simulink model "MinSegShield_Demo_M2V3"  (R2013a)
settings: Solver=FixedStepDiscrete  SolverMode=SingleTasking  StartTime=0.0  StopTime=inf  FixedStep=.1  RelTol=1e-3
libraries: arduinolib x5, MinSegLibrary_M2V3 x2
settings Model: SimulationMode=external  ExtModeTrigDuration=2  Creator=Alec  LastModifiedBy=hurstj
settings OptimizationCC: ExpressionDepthLimit=2147483647  OptimizeModelRefInitCode=on  LifeSpan=1
settings DebuggingCC: SolverPrmCheckMsg=none  StrictBusMsg=Warning
settings HardwareCC: ProdBitPerInt=16  ProdBitPerPointer=8  ProdIntDivRoundTo=Zero  ProdEndianess=LittleEndian  ProdWordSize=8  ProdHWDeviceType=Atmel->AVR
settings RTWCC: SystemTargetFile=realtime.tlc  GenerateMakefile=off  TemplateMakefile=realtime.tmf  Description=Real-Time Toolbox  RTWVerbose=off  ProcessScript=realtime_make_rtw_hook
settings CodeAppCC: CustomSymbolStrType=$N$R$M  InternalIdentifier=Classic
settings STFCustomTargetCC: TargetLibSuffix=.a  GenerateSampleERTMain=on  ERTCustomFileBanners=on  SupportNonInlinedSFcns=off  SupportVariableSizeSignals=on  MATLABClassNameForMDSCustomization=Simulink.SoftwareTarget.ERTCustomization  SystemTargetFile=realtime.tlc
settings ERTTargetCC: ParMdlRefBuildCompliant=off  CompOptLevelCompliant=off  ConcurrentExecutionCompliant=off  CombineOutputUpdateFcns=off  ERTFirstTimeCompliant=off  SupportContinuousTime=on  SupportVariableSizeSignals=on  ModelStepFunctionPrototypeControlCompliant=off  CPPClassGenCompliant=off  ExtMode=on  ExtModeTransport=3  ExtModeMexFile=ext_serial_win32_comm  ExtModeMexArgs=0 68 115200  ERTSrcFileBannerTemplate=realtime_code_template.cgt  ERTHdrFileBannerTemplate=realtime_code_template.cgt  ERTDataSrcFileTemplate=realtime_code_template.cgt  ERTDataHdrFileTemplate=realtime_code_template.cgt  ERTCustomFileTemplate=realtime_file_process.tlc

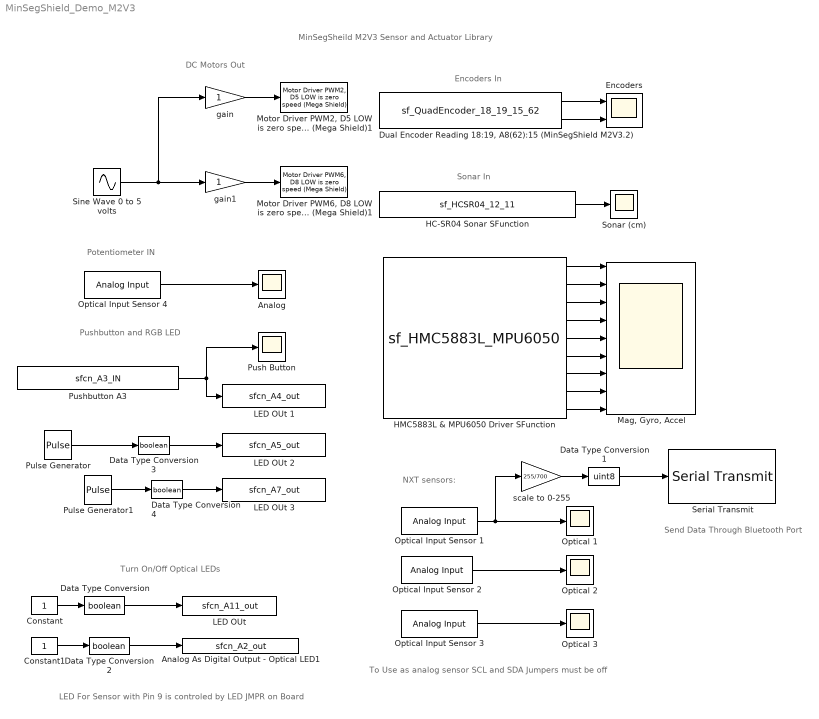
== system MinSegShield_Demo_M2V3 ==
  note: LED For Sensor with Pin 9
      |  is controled by LED JMPR on Board
  note: Turn On/Off Optical LEDs
  note: Send Data Through Bluetooth Port
  note: To Use as analog sensor SCL and SDA Jumpers must be off
  note: Potentiometer IN
  note: Pushbutton and RGB LED
  note: DC Motors Out
  note: Encoders In
  note: Sonar In
  note: NXT sensors:
  note: MinSegSheild M2V3 Sensor and Actuator Library
  Analog : Scope
      settings: TimeRange=30  YMin=0  YMax=1000  SaveName=ScopeData6
  Analog As Digital Output - Optical LED1 : S-Function  InitFcn=try, set_param(gcb,'FunctionName','sfcn_A2_out'), end  FunctionName=sfcn_A2_out  Parameters=uint8(12)  SFunctionModules=sfcn_A2_out_wrapper  EnableBusSupport=off  mask(S-Function Builder){}
      mask init:
      | val = [[.9  0.75 0.75 1 1 .9 .9 1]',[1 1 0.75 0.75 .9 .9 1 .9]'];try , sys = get_param(gcb,'SfunBuilderFcnName');if isempty(sys), sys = get_param(gcb,'FunctionName'); end,catch, sys = get_param(gcb,'FunctionName'); end
      settings: CopyFcn=set_param(gcbh,'LinkStatus','none')  PreSaveFcn=try, set_param(gcb,'FunctionName','sfcn_A2_out'), end  OpenFcn=sfunctionwizard(gcbh)
      mask Display: plot(val(:,1),val(:,2)),disp(sys), port_label('input',1,'in')
  Constant : Constant  SampleTime=-1
  Constant1 : Constant  SampleTime=-1
  Data Type Conversion{,2..4} (4 alike) : DataTypeConversion  OutDataTypeStr=boolean
  Data Type Conversion1 : DataTypeConversion  OutDataTypeStr=uint8
  "Dual Encoder Reading 18:19, A8(62):15 (MinSegShield M2V3.2) " : S-Function  InitFcn=try, set_param(gcb,'FunctionName','sf_QuadEncoder_18_19_15_62'), end  FunctionName=sf_QuadEncoder_18_19_15_62  Parameters=uint8([0 1]),uint8([18 62]),uint8([19 15])  SFunctionModules=sf_QuadEncoder_18_19_15_62_wrapper  EnableBusSupport=off  mask(S-Function Builder){}
      mask init: same as MinSegShield_Demo_M2V3/Analog As Digital Output - Optical LED1
      settings: CopyFcn=set_param(gcbh,'LinkStatus','none')  PreSaveFcn=try, set_param(gcb,'FunctionName','sf_QuadEncoder_18_19_15_62'), end  OpenFcn=sfunctionwizard(gcbh)
      mask Display: plot(val(:,1),val(:,2)),disp(sys), port_label('output',1,'pos1'), port_label('output',2,'pos2')
  Encoders : Scope  NumInputPorts=2
      settings: TimeRange=10  YMin=1700~-1500  YMax=2700~-500
  HC-SR04 Sonar SFunction : S-Function  InitFcn=try, set_param(gcb,'FunctionName','sf_HCSR04_12_11'), end  FunctionName=sf_HCSR04_12_11  SFunctionModules=sf_HCSR04_12_11_wrapper  EnableBusSupport=off  mask(S-Function Builder){}
      mask help: Simulink:masks:SFunctionBuilder_MD
      mask init: same as MinSegShield_Demo_M2V3/Analog As Digital Output - Optical LED1
      settings: CopyFcn=set_param(gcbh,'LinkStatus','none')  PreSaveFcn=try, set_param(gcb,'FunctionName','sf_HCSR04_12_11'), end  OpenFcn=sfunctionwizard(gcbh)
      mask Display:
      | plot(val(:,1),val(:,2))
      | disp(sys)
      | port_label('output',1,'distance_cm')
  HMC5883L & MPU6050 Driver SFunction : S-Function  InitFcn=try, set_param(gcb,'FunctionName','sf_HMC5883L_MPU6050'), end  FunctionName=sf_HMC5883L_MPU6050  SFunctionModules=sf_HMC5883L_MPU6050_wrapper  EnableBusSupport=off  mask(S-Function Builder){}
      mask help: Simulink:masks:SFunctionBuilder_MD
      mask init: same as MinSegShield_Demo_M2V3/Analog As Digital Output - Optical LED1
      settings: CopyFcn=set_param(gcbh,'LinkStatus','none')  PreSaveFcn=try, set_param(gcb,'FunctionName','sf_HMC5883L_MPU6050'), end  OpenFcn=sfunctionwizard(gcbh)
      mask Display:
      | plot(val(:,1),val(:,2))
      | disp(sys)
      | port_label('output',1,'x_mag')
      | port_label('output',2,'y_mag')
      | port_label('output',3,'z_mag')
      | port_label('output',4,'x_vel')
      | port_label('output',5,'y_vel')
      | port_label('output',6,'z_vel')
      | port_label('output',7,'x_acc')
      | port_label('output',8,'y_acc')
      | port_label('output',9,'z_acc')
  "LED OUt " : S-Function  InitFcn=try, set_param(gcb,'FunctionName','sfcn_A11_out'), end  FunctionName=sfcn_A11_out  Parameters=uint8(12)  SFunctionModules=sfcn_A11_out_wrapper  EnableBusSupport=off  mask(S-Function Builder){}
      mask init: same as MinSegShield_Demo_M2V3/Analog As Digital Output - Optical LED1
      settings: CopyFcn=set_param(gcbh,'LinkStatus','none')  PreSaveFcn=try, set_param(gcb,'FunctionName','sfcn_A11_out'), end  OpenFcn=sfunctionwizard(gcbh)
      mask Display: plot(val(:,1),val(:,2)),disp(sys), port_label('input',1,'in')
  LED OUt 1 : S-Function  InitFcn=try, set_param(gcb,'FunctionName','sfcn_A4_out'), end  FunctionName=sfcn_A4_out  Parameters=uint8(12)  SFunctionModules=sfcn_A4_out_wrapper  EnableBusSupport=off  mask(S-Function Builder){}
      mask init: same as MinSegShield_Demo_M2V3/Analog As Digital Output - Optical LED1
      settings: CopyFcn=set_param(gcbh,'LinkStatus','none')  PreSaveFcn=try, set_param(gcb,'FunctionName','sfcn_A4_out'), end  OpenFcn=sfunctionwizard(gcbh)
      mask Display: plot(val(:,1),val(:,2)),disp(sys), port_label('input',1,'in')
  LED OUt 2 : S-Function  InitFcn=try, set_param(gcb,'FunctionName','sfcn_A5_out'), end  FunctionName=sfcn_A5_out  Parameters=uint8(12)  SFunctionModules=sfcn_A5_out_wrapper  EnableBusSupport=off  mask(S-Function Builder){}
      mask init: same as MinSegShield_Demo_M2V3/Analog As Digital Output - Optical LED1
      settings: CopyFcn=set_param(gcbh,'LinkStatus','none')  PreSaveFcn=try, set_param(gcb,'FunctionName','sfcn_A5_out'), end  OpenFcn=sfunctionwizard(gcbh)
      mask Display: plot(val(:,1),val(:,2)),disp(sys), port_label('input',1,'in')
  LED OUt 3 : S-Function  InitFcn=try, set_param(gcb,'FunctionName','sfcn_A7_out'), end  FunctionName=sfcn_A7_out  Parameters=uint8(12)  SFunctionModules=sfcn_A7_out_wrapper  EnableBusSupport=off  mask(S-Function Builder){}
      mask init: same as MinSegShield_Demo_M2V3/Analog As Digital Output - Optical LED1
      settings: CopyFcn=set_param(gcbh,'LinkStatus','none')  PreSaveFcn=try, set_param(gcb,'FunctionName','sfcn_A7_out'), end  OpenFcn=sfunctionwizard(gcbh)
      mask Display: plot(val(:,1),val(:,2)),disp(sys), port_label('input',1,'in')
  "Mag, Gyro, Accel" : Scope  NumInputPorts=9
      settings: TimeRange=10  YMin=-15~-375~-80~-15000~-6000~-20000~-500~-12500~11000  YMax=20~-225~0~15000~5000~15000~3000~2500~20000
  "Motor Driver PWM2, D5 LOW is zero speed (Mega Shield)1" : MinSegLibrary_M2V3/Motor Driver PWM2, D5 LOW is zero speed (Mega Shield)
  "Motor Driver PWM6, D8 LOW is zero speed (Mega Shield)1" : MinSegLibrary_M2V3/Motor Driver PWM6, D8 LOW is zero speed (Mega Shield)
  Optical 1 : Scope
      settings: TimeRange=30  YMin=0  YMax=1000  SaveName=ScopeData4
  Optical 2 : Scope
      settings: TimeRange=30  YMin=0  YMax=1000  SaveName=ScopeData3
  Optical 3 : Scope
      settings: TimeRange=30  YMin=0  YMax=1000  SaveName=ScopeData5
  Optical Input Sensor 1 : arduinolib/Analog Input  pinNumber=10  sampleTime=-1
  Optical Input Sensor 2 : arduinolib/Analog Input  pinNumber=1  sampleTime=-1
  Optical Input Sensor 3 : arduinolib/Analog Input  pinNumber=9  sampleTime=-1
  Optical Input Sensor 4 : arduinolib/Analog Input  pinNumber=0  sampleTime=-1
  Pulse Generator : DiscretePulseGenerator  PulseType=Time based  Period=10  PulseWidth=50
  Pulse Generator1 : DiscretePulseGenerator  PulseType=Time based  Period=5  PulseWidth=50
  Push Button : Scope
      settings: TimeRange=30  YMin=0.95  YMax=1.05  SaveName=ScopeData7
  Pushbutton A3 : S-Function  InitFcn=try, set_param(gcb,'FunctionName','sfcn_A3_IN'), end  FunctionName=sfcn_A3_IN  SFunctionModules=sfcn_A3_IN_wrapper  EnableBusSupport=off  mask(S-Function Builder){}
      mask help: Simulink:masks:SFunctionBuilder_MD
      mask init: same as MinSegShield_Demo_M2V3/Analog As Digital Output - Optical LED1
      settings: CopyFcn=set_param(gcbh,'LinkStatus','none')  PreSaveFcn=try, set_param(gcb,'FunctionName','sfcn_A3_IN'), end  OpenFcn=sfunctionwizard(gcbh)
      mask Display: plot(val(:,1),val(:,2)),disp(sys), port_label('output',1,'push_button')
  Serial Transmit : arduinolib/Serial Transmit  portNumber=2
  Sine Wave 0 to 5 volts : Sin  SineType=Sample based  Amplitude=5  Frequency=50*2*pi  Samples=30  SampleTime=.1
  Sonar (cm) : Scope
      settings: TimeRange=10  YMin=0  YMax=175  SaveName=ScopeData2
  gain : Gain  OutDataTypeStr=int16
  gain1 : Gain  OutDataTypeStr=int16
  scale to 0-255 : Gain  Gain=255/700  OutDataTypeStr=int16
  wires:
  gain/1 -> "Motor Driver PWM2, D5 LOW is zero speed (Mega Shield)1"/1
  Sine Wave 0 to 5 volts/1 -> gain/1, gain1/1
  gain1/1 -> "Motor Driver PWM6, D8 LOW is zero speed (Mega Shield)1"/1
  "Dual Encoder Reading 18:19, A8(62):15 (MinSegShield M2V3.2) "/1 -> Encoders/1
  "Dual Encoder Reading 18:19, A8(62):15 (MinSegShield M2V3.2) "/2 -> Encoders/2
  HC-SR04 Sonar SFunction/1 -> Sonar (cm)/1
  Optical Input Sensor 1/1 -> scale to 0-255/1, Optical 1/1
  Constant/1 -> Data Type Conversion/1
  HMC5883L & MPU6050 Driver SFunction/1 -> "Mag, Gyro, Accel"/1
  HMC5883L & MPU6050 Driver SFunction/2 -> "Mag, Gyro, Accel"/2
  HMC5883L & MPU6050 Driver SFunction/3 -> "Mag, Gyro, Accel"/3
  HMC5883L & MPU6050 Driver SFunction/4 -> "Mag, Gyro, Accel"/4
  HMC5883L & MPU6050 Driver SFunction/5 -> "Mag, Gyro, Accel"/5
  HMC5883L & MPU6050 Driver SFunction/6 -> "Mag, Gyro, Accel"/6
  HMC5883L & MPU6050 Driver SFunction/7 -> "Mag, Gyro, Accel"/7
  HMC5883L & MPU6050 Driver SFunction/8 -> "Mag, Gyro, Accel"/8
  HMC5883L & MPU6050 Driver SFunction/9 -> "Mag, Gyro, Accel"/9
  scale to 0-255/1 -> Data Type Conversion1/1
  Data Type Conversion1/1 -> Serial Transmit/1
  Optical Input Sensor 2/1 -> Optical 2/1
  Optical Input Sensor 3/1 -> Optical 3/1
  Constant1/1 -> Data Type Conversion2/1
  Optical Input Sensor 4/1 -> Analog/1
  Pushbutton A3/1 -> LED OUt 1/1, Push Button/1
  Data Type Conversion/1 -> "LED OUt "/1
  Data Type Conversion2/1 -> Analog As Digital Output - Optical LED1/1
  Pulse Generator/1 -> Data Type Conversion3/1
  Pulse Generator1/1 -> Data Type Conversion4/1
  Data Type Conversion3/1 -> LED OUt 2/1
  Data Type Conversion4/1 -> LED OUt 3/1
